simulink library "inp"  (R2021b)
settings: Solver=VariableStepAuto  StartTime=0.0  StopTime=10.0  RelTol=1e-3
undefined symbols (not defined in the file): C_TASK_5MS_S, FALSE, KINP_AcoreReadyToSlp_flg_ovrdflg, KINP_AcoreReadyToSlp_flg_ovrdval, KINP_AllowMovThd_OTA_enum_ovrdflg, KINP_AllowMovThd_OTA_enum_ovrdval, KINP_APSAngleTarget_Deg_ovrdflg, KINP_APSAngleTarget_Deg_ovrdval, KINP_APSDecReq_mps2_ovrdflg, KINP_APSDecReq_mps2_ovrdval, KINP_APSDecReqA_flg_ovrdflg, KINP_APSDecReqA_flg_ovrdval, KINP_APSDFLL_cm_ovrdflg, KINP_APSDFLL_cm_ovrdval, KINP_APSDFLR_cm_ovrdflg, KINP_APSDFLR_cm_ovrdval, KINP_APSDRLL_cm_ovrdflg, KINP_APSDRLL_cm_ovrdval, KINP_APSDRLR_cm_ovrdflg, KINP_APSDRLR_cm_ovrdval, KINP_APSExitCondition_enum_ovrdflg, KINP_APSExitCondition_enum_ovrdval, KINP_APSHWVer_enum_ovrdflg, KINP_APSHWVer_enum_ovrdval, KINP_APSProgressPCT_pct_ovrdflg, KINP_APSProgressPCT_pct_ovrdval, KINP_APSReq_enum_ovrdflg, KINP_APSReq_enum_ovrdval, KINP_APSRQDisplay_enum_ovrdflg, KINP_APSRQDisplay_enum_ovrdval, KINP_APSRqEPASCtrl_flg_ovrdflg, KINP_APSRqEPASCtrl_flg_ovrdval, KINP_APSShiftPosnReq_enum_ovrdval, KINP_APSShiftPosnReq_enum_ovrflg, KINP_APSSpeedCMD_kph_ovrdval, KINP_APSSpeedCMD_kph_ovrflg, KINP_APSStaSystem_enum_ovrdflg, KINP_APSStaSystem_enum_ovrdval, KINP_APSSWVer_enum_ovrdflg, KINP_APSSWVer_enum_ovrdval, KINP_APSVMCReqA_flg_ovrdval, KINP_APSVMCReqA_flg_ovrflg, KINP_APSVRqEPASCtrl_flg_ovrdflg, KINP_APSVRqEPASCtrl_flg_ovrdval, KINP_AuxBattVolmV_mV_ovrdflg, KINP_AuxBattVolmV_mV_ovrdval, KINP_CAASSta_enum_ovrdflg, KINP_CAASSta_enum_ovrdval, KINP_CAASVMCReqA_flg_ovrdval, KINP_CAASVMCReqA_flg_ovrflg, KINP_Chime_enum_ovrdflg, KINP_Chime_enum_ovrdval, KINP_ClearDTCcmd_flg_ovrdflg, KINP_ClearDTCcmd_flg_ovrdval, KINP_EvccAplusPwrUpReq_flg_ovrdflg, KINP_EvccAplusPwrUpReq_flg_ovrdval, KINP_LFID_raw_ovrdval, KINP_LFID_raw_ovrflg, KINP_LRID_raw_ovrdval, KINP_MemOffsetAccX_raw16_ovrdflg ... (+118)
libraries: FVT_lib x942, hcu_lib x1
(part 4 of 31)

== system inp/INP/CAN2/CreateBus ==
  inp_CanValid_bus : Inport
  inp_Hal_bus : Inport  Port=2
  UnitConverter_{1..19,22..28,31,35,43..46,49..50,54,56..59,61,64,70..71,75..77,81,88,91..92,95..102,107..108,113,115..116,119..121,123,125,127..128,130,133..136,147,149,151,154,156..157,159,161,164,166} (85 alike) : DataTypeConversion  OutDataTypeStr=boolean
  UnitConverter_{37..42,48,65,103..106,109,117..118,122,137..142,144..145,168..169,171..172} (28 alike) : DataTypeConversion  OutDataTypeStr=single
  UnitConverter_{20..21,29..30,32..34,36,47,51..53,55,60,62..63,67..69,72..74,78..80,82..87,89..90,93..94,110..112,114,124,126,129,131..132,143,146,148,150,152..153,155,158,160,162..163,165,167,170} (58 alike) : DataTypeConversion  OutDataTypeStr=uint8
  UnitConverter_66 : DataTypeConversion  OutDataTypeStr=uint32
  bus_creator : BusCreator  Inputs=172
  bus_selector : BusSelector  OutputSignals=VINP_CANMsgValidHMI1_flg,VINP_CANMsgValidIVI1_flg,VINP_CANMsgValidIVI2_flg,VINP_CANMsgValidIVI3_flg,VINP_CANMsgValidMETER1_flg
  bus_selector_1 : BusSelector  OutputSignals=VINP_HMIACAirIntMCmd_flg,VINP_HMIACAirIntPCmd_flg,VINP_HMIACAutoBtnCmd_flg,VINP_HMIACBtnCmd_flg,VINP_HMIACFrDefogBtnCmd_flg,VINP_HMIACRecycleBtnCmd_flg,VINP_HMIACWindDirMCmd_flg,VINP_HMIACWindDirPCmd_flg,VINP_HMIZ1SetTMCmd_flg,VINP_HMIZ1SetTPCmd_flg,VINP_HMIZ2SetTMCmd_flg,VINP_HMIZ2SetTPCmd_flg,VINP_AmbLighLowBatAlertSW_flg,VINP_AmbLighSafetyAlertSW_flg,VINP_AmbLightBrightnessSet_enum,VINP_AmbLightColorSet_enum,VINP_AmbLightDimInDarkSW_flg,VINP_AmbLightSW_flg,VINP_AmbLightWlcmLightSW_flg,VINP_FCPFrEvtBtnACMaxReq_flg,VINP_FCPFrEvtBtnACReq_flg,VINP_FCPFrEvtBtnAutoReq_flg,VINP_FCPFrEvtBtnSyncReq_flg,VINP_IVICreateAccReqSta_enum,VINP_IVIDelAccReqSta_enum,VINP_IVILinkAccReqSta_flg,VINP_IVILinkAccSta_enum,VINP_IVILinkKeySta_enum,VINP_IVILocatedSTA_enum,VINP_IVILockSoundSWSta_flg,VINP_IVITimeCheck_enum,VINP_IVITimeDay_DAY,VINP_IVITimeHour_hr,VINP_IVITimeMinute_min,VINP_IVITimeMonth_MONTH,VINP_IVITimeSecond_s,VINP_IVITimeYear_YEAR,VINP_LINKtoDrive_flg,VINP_OpenDrOpenWdoSW_flg,VINP_PWCONTINUEUSE_flg,VINP_SmartEcoModeSW_flg,VINP_UserSet_enum,VINP_ACChgCurSet_A,VINP_AVMErrSTA_flg,VINP_AVMOFFRecButt_flg,VINP_AVMParkingmode_enum,VINP_AVMparkingcancel_enum,VINP_AVMparkingexcute_enum,VINP_ApproachUnlockSW_flg,VINP_CAASSw_enum,VINP_CDLLockButt_flg,VINP_CDLUnlockButt_flg,VINP_DSEATantiset_flg,VINP_DSEATentryfunset_flg,VINP_DSEATventreq_enum,VINP_Distanceunit_flg,VINP_ESCSWCmd_enum,VINP_FSOffSw_enum,VINP_FollowMeSW_flg,VINP_GPSLAT_s,VINP_GPSLONG_enum,VINP_HeadLampSW_enum,VINP_HoodLatchSW_enum,VINP_IVIAirIntZ3Cmd_enum,VINP_IVIChargePortSWSta_flg,VINP_IVICreepSWReq_flg,VINP_IVIDSEATHeaterCmd_enum,VINP_IVIDSEATFroEdgeHeightCmd_enum,VINP_IVIDSEATHeightCmd_enum,VINP_IVIDSEATMemory1Sta_flg,VINP_IVIDSEATMemory2Sta_flg,VINP_IVIDSEATMemoryOPTCLSSta_flg,VINP_IVIDSEATReclineCmd_enum,VINP_IVIDSEATSlideCmd_enum,VINP_IVIISAOffsetSpd_enum,VINP_IVINightModeSta_flg,VINP_IVIPSEATHeaterCmd_enum,VINP_IVIPSEATReclineCmd_enum,VINP_IVIPSEATSlideCmd_enum,VINP_IVIPTGModeSW_enum,VINP_IVIPTGOpenHeight_enum,VINP_IVIPTGStaSW_enum,VINP_IVIPTGUSStaSW_flg,VINP_IVIPWModeReq_enum,VINP_IVIPwrLockSW_enum,VINP_IVIPwroffreq_flg,VINP_IVIRRDefReq_flg,VINP_IVIReqV2L_enum,VINP_IVIScreen_enum,VINP_IVIStartChgreq_flg,VINP_IVIStatus_flg,VINP_IVIStopChgreq_flg,VINP_IVITrailerCheckReqSta_flg,VINP_IVITrailerModeSWSta_flg,VINP_IVITriggerreq_flg,VINP_IVIUnlockChgreq_flg,VINP_IVIWIMAINSW_flg,VINP_LDrvControlCommand_pct,VINP_LPasControlCommand_pct,VINP_LRLDControlCommand_pct,VINP_LRRDControlCommand_pct,VINP_LightShowStartReq_flg,VINP_LightShowStopReq_flg,VINP_MFRDNBrightReq_pct,VINP_OFFACMODE_enum,VINP_PSEATventreq_enum,VINP_PerdV2L_enum,VINP_RFogLampSW_flg,VINP_RollModeSWCmd_enum,VINP_RoomLampMode_flg,VINP_SOCADJBUTT_flg,VINP_SOCLimitSet_pct,VINP_SOCV2LLimit_pct,VINP_SchedChgStart_flg,VINP_SchedChgStop_flg,VINP_SchedChgbutt_flg,VINP_SchedChglimit_pct,VINP_SchedChgwake_flg,VINP_SenstivityPosition_enum,VINP_SetUnlockSingle_flg,VINP_TCSSWCmd_enum,VINP_TPMSCaliButt_flg,VINP_TPMSResButt_flg,VINP_TurnSwTimeSet_enum,VINP_WalkawayLockSW_flg,VINP_WlcmLightMode_enum,VINP_sigAirIntenZon1Req_enum,VINP_sigDfrstReq_flg,VINP_sigFaceReq_flg,VINP_sigFootReq_flg,VINP_sigRecircReq_flg,VINP_sigSetTempZon1Req_C,VINP_sigSetTempZon2Req_C,VINP_IVICLBlowerYSta_pct,VINP_IVICLBlowerZSta_pct,VINP_IVICRBlowerYSta_pct,VINP_IVICRBlowerZSta_pct,VINP_IVIDrBlowerModeSta_enum,VINP_IVIDrBlowerYSta_pct,VINP_IVIDrBlowerZSta_pct,VINP_IVILSEATventCmd_enum,VINP_IVIMLFMostCmd_flg,VINP_IVIMLFootLiftCmd_enum,VINP_IVIMLNapModeCmd_flg,VINP_IVIMLReclinerCmd_enum,VINP_IVIMLRestoreCmd_flg,VINP_IVIMLSEATventCmd_enum,VINP_IVIMLSeatLiftCmd_enum,VINP_IVIMLSldRestoreCmd_flg,VINP_IVIMLSliderCmd_enum,VINP_IVIMLZeroGravityCmd_flg,VINP_IVIMRFMostCmd_flg,VINP_IVIMRFootLiftCmd_enum,VINP_IVIMRNapModeCmd_flg,VINP_IVIMRReclinerCmd_enum,VINP_IVIMRRestoreCmd_flg,VINP_IVIMRSEATventCmd_enum,VINP_IVIMRSeatLiftCmd_enum,VINP_IVIMRSldRestoreCmd_flg,VINP_IVIMRSliderCmd_enum,VINP_IVIMRZeroGravityCmd_flg,VINP_IVIPsBlowerModeSta_enum,VINP_IVIPsBlowerYSta_pct,VINP_IVIPsBlowerZSta_pct,VINP_IVIRSEATventCmd_enum,VINP_METERKPHCalcu_kph,VINP_ODOMETER_km
  BINP_outputs : Outport
  wires:
  inp_CanValid_bus/1 -> [inp_CanValid_bus]
  inp_Hal_bus/1 -> [inp_Hal_bus]
  bus_selector/1 -> UnitConverter_1/1  "<VINP_CANMsgValidHMI1_flg>"
  UnitConverter_1/1 -> bus_creator/1  "VINP_CANMsgValidHMI1_flg"
  bus_selector/2 -> UnitConverter_2/1  "<VINP_CANMsgValidIVI1_flg>"
  UnitConverter_2/1 -> bus_creator/2  "VINP_CANMsgValidIVI1_flg"
  bus_selector/3 -> UnitConverter_3/1  "<VINP_CANMsgValidIVI2_flg>"
  UnitConverter_3/1 -> bus_creator/3  "VINP_CANMsgValidIVI2_flg"
  bus_selector/4 -> UnitConverter_4/1  "<VINP_CANMsgValidIVI3_flg>"
  UnitConverter_4/1 -> bus_creator/4  "VINP_CANMsgValidIVI3_flg"
  bus_selector/5 -> UnitConverter_5/1  "<VINP_CANMsgValidMETER1_flg>"
  UnitConverter_5/1 -> bus_creator/5  "VINP_CANMsgValidMETER1_flg"
  bus_selector_1/1 -> UnitConverter_6/1  "<VINP_HMIACAirIntMCmd_flg>"
  UnitConverter_6/1 -> bus_creator/6  "VINP_HMIACAirIntMCmd_flg"
  bus_selector_1/2 -> UnitConverter_7/1  "<VINP_HMIACAirIntPCmd_flg>"
  UnitConverter_7/1 -> bus_creator/7  "VINP_HMIACAirIntPCmd_flg"
  bus_selector_1/3 -> UnitConverter_8/1  "<VINP_HMIACAutoBtnCmd_flg>"
  UnitConverter_8/1 -> bus_creator/8  "VINP_HMIACAutoBtnCmd_flg"
  bus_selector_1/4 -> UnitConverter_9/1  "<VINP_HMIACBtnCmd_flg>"
  UnitConverter_9/1 -> bus_creator/9  "VINP_HMIACBtnCmd_flg"
  bus_selector_1/5 -> UnitConverter_10/1  "<VINP_HMIACFrDefogBtnCmd_flg>"
  UnitConverter_10/1 -> bus_creator/10  "VINP_HMIACFrDefogBtnCmd_flg"
  bus_selector_1/6 -> UnitConverter_11/1  "<VINP_HMIACRecycleBtnCmd_flg>"
  UnitConverter_11/1 -> bus_creator/11  "VINP_HMIACRecycleBtnCmd_flg"
  bus_selector_1/7 -> UnitConverter_12/1  "<VINP_HMIACWindDirMCmd_flg>"
  UnitConverter_12/1 -> bus_creator/12  "VINP_HMIACWindDirMCmd_flg"
  bus_selector_1/8 -> UnitConverter_13/1  "<VINP_HMIACWindDirPCmd_flg>"
  UnitConverter_13/1 -> bus_creator/13  "VINP_HMIACWindDirPCmd_flg"
  bus_selector_1/9 -> UnitConverter_14/1  "<VINP_HMIZ1SetTMCmd_flg>"
  UnitConverter_14/1 -> bus_creator/14  "VINP_HMIZ1SetTMCmd_flg"
  bus_selector_1/10 -> UnitConverter_15/1  "<VINP_HMIZ1SetTPCmd_flg>"
  UnitConverter_15/1 -> bus_creator/15  "VINP_HMIZ1SetTPCmd_flg"
  bus_selector_1/11 -> UnitConverter_16/1  "<VINP_HMIZ2SetTMCmd_flg>"
  UnitConverter_16/1 -> bus_creator/16  "VINP_HMIZ2SetTMCmd_flg"
  bus_selector_1/12 -> UnitConverter_17/1  "<VINP_HMIZ2SetTPCmd_flg>"
  UnitConverter_17/1 -> bus_creator/17  "VINP_HMIZ2SetTPCmd_flg"
  bus_selector_1/13 -> UnitConverter_18/1  "<VINP_AmbLighLowBatAlertSW_flg>"
  UnitConverter_18/1 -> bus_creator/18  "VINP_AmbLighLowBatAlertSW_flg"
  bus_selector_1/14 -> UnitConverter_19/1  "<VINP_AmbLighSafetyAlertSW_flg>"
  UnitConverter_19/1 -> bus_creator/19  "VINP_AmbLighSafetyAlertSW_flg"
  bus_selector_1/15 -> UnitConverter_20/1  "<VINP_AmbLightBrightnessSet_enum>"
  UnitConverter_20/1 -> bus_creator/20  "VINP_AmbLightBrightnessSet_enum"
  bus_selector_1/16 -> UnitConverter_21/1  "<VINP_AmbLightColorSet_enum>"
  UnitConverter_21/1 -> bus_creator/21  "VINP_AmbLightColorSet_enum"
  bus_selector_1/17 -> UnitConverter_22/1  "<VINP_AmbLightDimInDarkSW_flg>"
  UnitConverter_22/1 -> bus_creator/22  "VINP_AmbLightDimInDarkSW_flg"
  bus_selector_1/18 -> UnitConverter_23/1  "<VINP_AmbLightSW_flg>"
  UnitConverter_23/1 -> bus_creator/23  "VINP_AmbLightSW_flg"
  bus_selector_1/19 -> UnitConverter_24/1  "<VINP_AmbLightWlcmLightSW_flg>"
  UnitConverter_24/1 -> bus_creator/24  "VINP_AmbLightWlcmLightSW_flg"
  bus_selector_1/20 -> UnitConverter_25/1  "<VINP_FCPFrEvtBtnACMaxReq_flg>"
  UnitConverter_25/1 -> bus_creator/25  "VINP_FCPFrEvtBtnACMaxReq_flg"
  bus_selector_1/21 -> UnitConverter_26/1  "<VINP_FCPFrEvtBtnACReq_flg>"
  UnitConverter_26/1 -> bus_creator/26  "VINP_FCPFrEvtBtnACReq_flg"
  bus_selector_1/22 -> UnitConverter_27/1  "<VINP_FCPFrEvtBtnAutoReq_flg>"
  UnitConverter_27/1 -> bus_creator/27  "VINP_FCPFrEvtBtnAutoReq_flg"
  bus_selector_1/23 -> UnitConverter_28/1  "<VINP_FCPFrEvtBtnSyncReq_flg>"
  UnitConverter_28/1 -> bus_creator/28  "VINP_FCPFrEvtBtnSyncReq_flg"
  bus_selector_1/24 -> UnitConverter_29/1  "<VINP_IVICreateAccReqSta_enum>"
  UnitConverter_29/1 -> bus_creator/29  "VINP_IVICreateAccReqSta_enum"
  bus_selector_1/25 -> UnitConverter_30/1  "<VINP_IVIDelAccReqSta_enum>"
  UnitConverter_30/1 -> bus_creator/30  "VINP_IVIDelAccReqSta_enum"
  bus_selector_1/26 -> UnitConverter_31/1  "<VINP_IVILinkAccReqSta_flg>"
  UnitConverter_31/1 -> bus_creator/31  "VINP_IVILinkAccReqSta_flg"
  bus_selector_1/27 -> UnitConverter_32/1  "<VINP_IVILinkAccSta_enum>"
  UnitConverter_32/1 -> bus_creator/32  "VINP_IVILinkAccSta_enum"
  bus_selector_1/28 -> UnitConverter_33/1  "<VINP_IVILinkKeySta_enum>"
  UnitConverter_33/1 -> bus_creator/33  "VINP_IVILinkKeySta_enum"
  bus_selector_1/29 -> UnitConverter_34/1  "<VINP_IVILocatedSTA_enum>"
  UnitConverter_34/1 -> bus_creator/34  "VINP_IVILocatedSTA_enum"
  bus_selector_1/30 -> UnitConverter_35/1  "<VINP_IVILockSoundSWSta_flg>"
  UnitConverter_35/1 -> bus_creator/35  "VINP_IVILockSoundSWSta_flg"
  bus_selector_1/31 -> UnitConverter_36/1  "<VINP_IVITimeCheck_enum>"
  UnitConverter_36/1 -> bus_creator/36  "VINP_IVITimeCheck_enum"
  bus_selector_1/32 -> UnitConverter_37/1  "<VINP_IVITimeDay_DAY>"
  UnitConverter_37/1 -> bus_creator/37  "VINP_IVITimeDay_DAY"
  bus_selector_1/33 -> UnitConverter_38/1  "<VINP_IVITimeHour_hr>"
  UnitConverter_38/1 -> bus_creator/38  "VINP_IVITimeHour_hr"
  bus_selector_1/34 -> UnitConverter_39/1  "<VINP_IVITimeMinute_min>"
  UnitConverter_39/1 -> bus_creator/39  "VINP_IVITimeMinute_min"
  bus_selector_1/35 -> UnitConverter_40/1  "<VINP_IVITimeMonth_MONTH>"
  UnitConverter_40/1 -> bus_creator/40  "VINP_IVITimeMonth_MONTH"
  bus_selector_1/36 -> UnitConverter_41/1  "<VINP_IVITimeSecond_s>"
  UnitConverter_41/1 -> bus_creator/41  "VINP_IVITimeSecond_s"
  bus_selector_1/37 -> UnitConverter_42/1  "<VINP_IVITimeYear_YEAR>"
  UnitConverter_42/1 -> bus_creator/42  "VINP_IVITimeYear_YEAR"
  bus_selector_1/38 -> UnitConverter_43/1  "<VINP_LINKtoDrive_flg>"
  UnitConverter_43/1 -> bus_creator/43  "VINP_LINKtoDrive_flg"
  bus_selector_1/39 -> UnitConverter_44/1  "<VINP_OpenDrOpenWdoSW_flg>"
  UnitConverter_44/1 -> bus_creator/44  "VINP_OpenDrOpenWdoSW_flg"
  bus_selector_1/40 -> UnitConverter_45/1  "<VINP_PWCONTINUEUSE_flg>"
  UnitConverter_45/1 -> bus_creator/45  "VINP_PWCONTINUEUSE_flg"
  bus_selector_1/41 -> UnitConverter_46/1  "<VINP_SmartEcoModeSW_flg>"
  UnitConverter_46/1 -> bus_creator/46  "VINP_SmartEcoModeSW_flg"
  bus_selector_1/42 -> UnitConverter_47/1  "<VINP_UserSet_enum>"
  UnitConverter_47/1 -> bus_creator/47  "VINP_UserSet_enum"
  bus_selector_1/43 -> UnitConverter_48/1  "<VINP_ACChgCurSet_A>"
  UnitConverter_48/1 -> bus_creator/48  "VINP_ACChgCurSet_A"
  bus_selector_1/44 -> UnitConverter_49/1  "<VINP_AVMErrSTA_flg>"
  UnitConverter_49/1 -> bus_creator/49  "VINP_AVMErrSTA_flg"
  bus_selector_1/45 -> UnitConverter_50/1  "<VINP_AVMOFFRecButt_flg>"
  UnitConverter_50/1 -> bus_creator/50  "VINP_AVMOFFRecButt_flg"
  bus_selector_1/46 -> UnitConverter_51/1  "<VINP_AVMParkingmode_enum>"
  UnitConverter_51/1 -> bus_creator/51  "VINP_AVMParkingmode_enum"
  bus_selector_1/47 -> UnitConverter_52/1  "<VINP_AVMparkingcancel_enum>"
  UnitConverter_52/1 -> bus_creator/52  "VINP_AVMparkingcancel_enum"
  bus_selector_1/48 -> UnitConverter_53/1  "<VINP_AVMparkingexcute_enum>"
  UnitConverter_53/1 -> bus_creator/53  "VINP_AVMparkingexcute_enum"
  bus_selector_1/49 -> UnitConverter_54/1  "<VINP_ApproachUnlockSW_flg>"
  UnitConverter_54/1 -> bus_creator/54  "VINP_ApproachUnlockSW_flg"
  bus_selector_1/50 -> UnitConverter_55/1  "<VINP_CAASSw_enum>"
  UnitConverter_55/1 -> bus_creator/55  "VINP_CAASSw_enum"
  bus_selector_1/51 -> UnitConverter_56/1  "<VINP_CDLLockButt_flg>"
  UnitConverter_56/1 -> bus_creator/56  "VINP_CDLLockButt_flg"
  bus_selector_1/52 -> UnitConverter_57/1  "<VINP_CDLUnlockButt_flg>"
  UnitConverter_57/1 -> bus_creator/57  "VINP_CDLUnlockButt_flg"
  bus_selector_1/53 -> UnitConverter_58/1  "<VINP_DSEATantiset_flg>"
  UnitConverter_58/1 -> bus_creator/58  "VINP_DSEATantiset_flg"
  bus_selector_1/54 -> UnitConverter_59/1  "<VINP_DSEATentryfunset_flg>"
  UnitConverter_59/1 -> bus_creator/59  "VINP_DSEATentryfunset_flg"
  bus_selector_1/55 -> UnitConverter_60/1  "<VINP_DSEATventreq_enum>"
  UnitConverter_60/1 -> bus_creator/60  "VINP_DSEATventreq_enum"
  bus_selector_1/56 -> UnitConverter_61/1  "<VINP_Distanceunit_flg>"
  UnitConverter_61/1 -> bus_creator/61  "VINP_Distanceunit_flg"
  bus_selector_1/57 -> UnitConverter_62/1  "<VINP_ESCSWCmd_enum>"
  UnitConverter_62/1 -> bus_creator/62  "VINP_ESCSWCmd_enum"
  bus_selector_1/58 -> UnitConverter_63/1  "<VINP_FSOffSw_enum>"
  UnitConverter_63/1 -> bus_creator/63  "VINP_FSOffSw_enum"
  bus_selector_1/59 -> UnitConverter_64/1  "<VINP_FollowMeSW_flg>"
  UnitConverter_64/1 -> bus_creator/64  "VINP_FollowMeSW_flg"
  bus_selector_1/60 -> UnitConverter_65/1  "<VINP_GPSLAT_s>"
  UnitConverter_65/1 -> bus_creator/65  "VINP_GPSLAT_s"
  bus_selector_1/61 -> UnitConverter_66/1  "<VINP_GPSLONG_enum>"
  UnitConverter_66/1 -> bus_creator/66  "VINP_GPSLONG_enum"
  bus_selector_1/62 -> UnitConverter_67/1  "<VINP_HeadLampSW_enum>"
  UnitConverter_67/1 -> bus_creator/67  "VINP_HeadLampSW_enum"
  bus_selector_1/63 -> UnitConverter_68/1  "<VINP_HoodLatchSW_enum>"
  UnitConverter_68/1 -> bus_creator/68  "VINP_HoodLatchSW_enum"
  bus_selector_1/64 -> UnitConverter_69/1  "<VINP_IVIAirIntZ3Cmd_enum>"
  UnitConverter_69/1 -> bus_creator/69  "VINP_IVIAirIntZ3Cmd_enum"
  bus_selector_1/65 -> UnitConverter_70/1  "<VINP_IVIChargePortSWSta_flg>"
  UnitConverter_70/1 -> bus_creator/70  "VINP_IVIChargePortSWSta_flg"
  bus_selector_1/66 -> UnitConverter_71/1  "<VINP_IVICreepSWReq_flg>"
  UnitConverter_71/1 -> bus_creator/71  "VINP_IVICreepSWReq_flg"
  bus_selector_1/67 -> UnitConverter_72/1  "<VINP_IVIDSEATHeaterCmd_enum>"
  UnitConverter_72/1 -> bus_creator/72  "VINP_IVIDSEATHeaterCmd_enum"
  bus_selector_1/68 -> UnitConverter_73/1  "<VINP_IVIDSEATFroEdgeHeightCmd_enum>"
  UnitConverter_73/1 -> bus_creator/73  "VINP_IVIDSEATFroEdgeHeightCmd_enum"
  bus_selector_1/69 -> UnitConverter_74/1  "<VINP_IVIDSEATHeightCmd_enum>"
  UnitConverter_74/1 -> bus_creator/74  "VINP_IVIDSEATHeightCmd_enum"
  bus_selector_1/70 -> UnitConverter_75/1  "<VINP_IVIDSEATMemory1Sta_flg>"
  UnitConverter_75/1 -> bus_creator/75  "VINP_IVIDSEATMemory1Sta_flg"
  bus_selector_1/71 -> UnitConverter_76/1  "<VINP_IVIDSEATMemory2Sta_flg>"
  UnitConverter_76/1 -> bus_creator/76  "VINP_IVIDSEATMemory2Sta_flg"
  bus_selector_1/72 -> UnitConverter_77/1  "<VINP_IVIDSEATMemoryOPTCLSSta_flg>"
  UnitConverter_77/1 -> bus_creator/77  "VINP_IVIDSEATMemoryOPTCLSSta_flg"
  bus_selector_1/73 -> UnitConverter_78/1  "<VINP_IVIDSEATReclineCmd_enum>"
  UnitConverter_78/1 -> bus_creator/78  "VINP_IVIDSEATReclineCmd_enum"
  bus_selector_1/74 -> UnitConverter_79/1  "<VINP_IVIDSEATSlideCmd_enum>"
  UnitConverter_79/1 -> bus_creator/79  "VINP_IVIDSEATSlideCmd_enum"
  bus_selector_1/75 -> UnitConverter_80/1  "<VINP_IVIISAOffsetSpd_enum>"
  UnitConverter_80/1 -> bus_creator/80  "VINP_IVIISAOffsetSpd_enum"
  bus_selector_1/76 -> UnitConverter_81/1  "<VINP_IVINightModeSta_flg>"
  UnitConverter_81/1 -> bus_creator/81  "VINP_IVINightModeSta_flg"
  bus_selector_1/77 -> UnitConverter_82/1  "<VINP_IVIPSEATHeaterCmd_enum>"
  UnitConverter_82/1 -> bus_creator/82  "VINP_IVIPSEATHeaterCmd_enum"
  bus_selector_1/78 -> UnitConverter_83/1  "<VINP_IVIPSEATReclineCmd_enum>"
  UnitConverter_83/1 -> bus_creator/83  "VINP_IVIPSEATReclineCmd_enum"
  bus_selector_1/79 -> UnitConverter_84/1  "<VINP_IVIPSEATSlideCmd_enum>"
  UnitConverter_84/1 -> bus_creator/84  "VINP_IVIPSEATSlideCmd_enum"
  bus_selector_1/80 -> UnitConverter_85/1  "<VINP_IVIPTGModeSW_enum>"
  UnitConverter_85/1 -> bus_creator/85  "VINP_IVIPTGModeSW_enum"
  bus_selector_1/81 -> UnitConverter_86/1  "<VINP_IVIPTGOpenHeight_enum>"
  UnitConverter_86/1 -> bus_creator/86  "VINP_IVIPTGOpenHeight_enum"
  bus_selector_1/82 -> UnitConverter_87/1  "<VINP_IVIPTGStaSW_enum>"
  UnitConverter_87/1 -> bus_creator/87  "VINP_IVIPTGStaSW_enum"
  bus_selector_1/83 -> UnitConverter_88/1  "<VINP_IVIPTGUSStaSW_flg>"
  UnitConverter_88/1 -> bus_creator/88  "VINP_IVIPTGUSStaSW_flg"
  bus_selector_1/84 -> UnitConverter_89/1  "<VINP_IVIPWModeReq_enum>"
  UnitConverter_89/1 -> bus_creator/89  "VINP_IVIPWModeReq_enum"
  bus_selector_1/85 -> UnitConverter_90/1  "<VINP_IVIPwrLockSW_enum>"
  UnitConverter_90/1 -> bus_creator/90  "VINP_IVIPwrLockSW_enum"
  bus_selector_1/86 -> UnitConverter_91/1  "<VINP_IVIPwroffreq_flg>"
  UnitConverter_91/1 -> bus_creator/91  "VINP_IVIPwroffreq_flg"
  bus_selector_1/87 -> UnitConverter_92/1  "<VINP_IVIRRDefReq_flg>"
  UnitConverter_92/1 -> bus_creator/92  "VINP_IVIRRDefReq_flg"
  bus_selector_1/88 -> UnitConverter_93/1  "<VINP_IVIReqV2L_enum>"
  UnitConverter_93/1 -> bus_creator/93  "VINP_IVIReqV2L_enum"
  bus_selector_1/89 -> UnitConverter_94/1  "<VINP_IVIScreen_enum>"
  UnitConverter_94/1 -> bus_creator/94  "VINP_IVIScreen_enum"
  bus_selector_1/90 -> UnitConverter_95/1  "<VINP_IVIStartChgreq_flg>"
  UnitConverter_95/1 -> bus_creator/95  "VINP_IVIStartChgreq_flg"
  bus_selector_1/91 -> UnitConverter_96/1  "<VINP_IVIStatus_flg>"
  UnitConverter_96/1 -> bus_creator/96  "VINP_IVIStatus_flg"
  bus_selector_1/92 -> UnitConverter_97/1  "<VINP_IVIStopChgreq_flg>"
  UnitConverter_97/1 -> bus_creator/97  "VINP_IVIStopChgreq_flg"
  bus_selector_1/93 -> UnitConverter_98/1  "<VINP_IVITrailerCheckReqSta_flg>"
  UnitConverter_98/1 -> bus_creator/98  "VINP_IVITrailerCheckReqSta_flg"
  bus_selector_1/94 -> UnitConverter_99/1  "<VINP_IVITrailerModeSWSta_flg>"
  UnitConverter_99/1 -> bus_creator/99  "VINP_IVITrailerModeSWSta_flg"
  bus_selector_1/95 -> UnitConverter_100/1  "<VINP_IVITriggerreq_flg>"
  UnitConverter_100/1 -> bus_creator/100  "VINP_IVITriggerreq_flg"
  bus_selector_1/96 -> UnitConverter_101/1  "<VINP_IVIUnlockChgreq_flg>"
  UnitConverter_101/1 -> bus_creator/101  "VINP_IVIUnlockChgreq_flg"
  bus_selector_1/97 -> UnitConverter_102/1  "<VINP_IVIWIMAINSW_flg>"
  UnitConverter_102/1 -> bus_creator/102  "VINP_IVIWIMAINSW_flg"
  bus_selector_1/98 -> UnitConverter_103/1  "<VINP_LDrvControlCommand_pct>"
  UnitConverter_103/1 -> bus_creator/103  "VINP_LDrvControlCommand_pct"
  bus_selector_1/99 -> UnitConverter_104/1  "<VINP_LPasControlCommand_pct>"
  UnitConverter_104/1 -> bus_creator/104  "VINP_LPasControlCommand_pct"
  bus_selector_1/100 -> UnitConverter_105/1  "<VINP_LRLDControlCommand_pct>"
  UnitConverter_105/1 -> bus_creator/105  "VINP_LRLDControlCommand_pct"
  bus_selector_1/101 -> UnitConverter_106/1  "<VINP_LRRDControlCommand_pct>"
  UnitConverter_106/1 -> bus_creator/106  "VINP_LRRDControlCommand_pct"
  bus_selector_1/102 -> UnitConverter_107/1  "<VINP_LightShowStartReq_flg>"
  UnitConverter_107/1 -> bus_creator/107  "VINP_LightShowStartReq_flg"
  bus_selector_1/103 -> UnitConverter_108/1  "<VINP_LightShowStopReq_flg>"
  UnitConverter_108/1 -> bus_creator/108  "VINP_LightShowStopReq_flg"
  bus_selector_1/104 -> UnitConverter_109/1  "<VINP_MFRDNBrightReq_pct>"
  UnitConverter_109/1 -> bus_creator/109  "VINP_MFRDNBrightReq_pct"
  bus_selector_1/105 -> UnitConverter_110/1  "<VINP_OFFACMODE_enum>"
  UnitConverter_110/1 -> bus_creator/110  "VINP_OFFACMODE_enum"
  bus_selector_1/106 -> UnitConverter_111/1  "<VINP_PSEATventreq_enum>"
  UnitConverter_111/1 -> bus_creator/111  "VINP_PSEATventreq_enum"
  bus_selector_1/107 -> UnitConverter_112/1  "<VINP_PerdV2L_enum>"
  UnitConverter_112/1 -> bus_creator/112  "VINP_PerdV2L_enum"
  bus_selector_1/108 -> UnitConverter_113/1  "<VINP_RFogLampSW_flg>"
  UnitConverter_113/1 -> bus_creator/113  "VINP_RFogLampSW_flg"
  bus_selector_1/109 -> UnitConverter_114/1  "<VINP_RollModeSWCmd_enum>"
  UnitConverter_114/1 -> bus_creator/114  "VINP_RollModeSWCmd_enum"
  bus_selector_1/110 -> UnitConverter_115/1  "<VINP_RoomLampMode_flg>"
  UnitConverter_115/1 -> bus_creator/115  "VINP_RoomLampMode_flg"
  bus_selector_1/111 -> UnitConverter_116/1  "<VINP_SOCADJBUTT_flg>"
  UnitConverter_116/1 -> bus_creator/116  "VINP_SOCADJBUTT_flg"
  bus_selector_1/112 -> UnitConverter_117/1  "<VINP_SOCLimitSet_pct>"
  UnitConverter_117/1 -> bus_creator/117  "VINP_SOCLimitSet_pct"
  bus_selector_1/113 -> UnitConverter_118/1  "<VINP_SOCV2LLimit_pct>"
  UnitConverter_118/1 -> bus_creator/118  "VINP_SOCV2LLimit_pct"
  bus_selector_1/114 -> UnitConverter_119/1  "<VINP_SchedChgStart_flg>"
  UnitConverter_119/1 -> bus_creator/119  "VINP_SchedChgStart_flg"
  bus_selector_1/115 -> UnitConverter_120/1  "<VINP_SchedChgStop_flg>"
  UnitConverter_120/1 -> bus_creator/120  "VINP_SchedChgStop_flg"
  bus_selector_1/116 -> UnitConverter_121/1  "<VINP_SchedChgbutt_flg>"
  UnitConverter_121/1 -> bus_creator/121  "VINP_SchedChgbutt_flg"
  bus_selector_1/117 -> UnitConverter_122/1  "<VINP_SchedChglimit_pct>"
  UnitConverter_122/1 -> bus_creator/122  "VINP_SchedChglimit_pct"
  bus_selector_1/118 -> UnitConverter_123/1  "<VINP_SchedChgwake_flg>"
  UnitConverter_123/1 -> bus_creator/123  "VINP_SchedChgwake_flg"
  bus_selector_1/119 -> UnitConverter_124/1  "<VINP_SenstivityPosition_enum>"
  UnitConverter_124/1 -> bus_creator/124  "VINP_SenstivityPosition_enum"
  bus_selector_1/120 -> UnitConverter_125/1  "<VINP_SetUnlockSingle_flg>"
  UnitConverter_125/1 -> bus_creator/125  "VINP_SetUnlockSingle_flg"
  bus_selector_1/121 -> UnitConverter_126/1  "<VINP_TCSSWCmd_enum>"
  UnitConverter_126/1 -> bus_creator/126  "VINP_TCSSWCmd_enum"
  bus_selector_1/122 -> UnitConverter_127/1  "<VINP_TPMSCaliButt_flg>"
  UnitConverter_127/1 -> bus_creator/127  "VINP_TPMSCaliButt_flg"
  bus_selector_1/123 -> UnitConverter_128/1  "<VINP_TPMSResButt_flg>"
  UnitConverter_128/1 -> bus_creator/128  "VINP_TPMSResButt_flg"
  bus_selector_1/124 -> UnitConverter_129/1  "<VINP_TurnSwTimeSet_enum>"
  UnitConverter_129/1 -> bus_creator/129  "VINP_TurnSwTimeSet_enum"
  bus_selector_1/125 -> UnitConverter_130/1  "<VINP_WalkawayLockSW_flg>"
  UnitConverter_130/1 -> bus_creator/130  "VINP_WalkawayLockSW_flg"
  bus_selector_1/126 -> UnitConverter_131/1  "<VINP_WlcmLightMode_enum>"
  UnitConverter_131/1 -> bus_creator/131  "VINP_WlcmLightMode_enum"
  bus_selector_1/127 -> UnitConverter_132/1  "<VINP_sigAirIntenZon1Req_enum>"
  UnitConverter_132/1 -> bus_creator/132  "VINP_sigAirIntenZon1Req_enum"
  bus_selector_1/128 -> UnitConverter_133/1  "<VINP_sigDfrstReq_flg>"
  UnitConverter_133/1 -> bus_creator/133  "VINP_sigDfrstReq_flg"
  bus_selector_1/129 -> UnitConverter_134/1  "<VINP_sigFaceReq_flg>"
  UnitConverter_134/1 -> bus_creator/134  "VINP_sigFaceReq_flg"
  bus_selector_1/130 -> UnitConverter_135/1  "<VINP_sigFootReq_flg>"
  UnitConverter_135/1 -> bus_creator/135  "VINP_sigFootReq_flg"
  bus_selector_1/131 -> UnitConverter_136/1  "<VINP_sigRecircReq_flg>"
  UnitConverter_136/1 -> bus_creator/136  "VINP_sigRecircReq_flg"
  bus_selector_1/132 -> UnitConverter_137/1  "<VINP_sigSetTempZon1Req_C>"
  UnitConverter_137/1 -> bus_creator/137  "VINP_sigSetTempZon1Req_C"
  bus_selector_1/133 -> UnitConverter_138/1  "<VINP_sigSetTempZon2Req_C>"
  UnitConverter_138/1 -> bus_creator/138  "VINP_sigSetTempZon2Req_C"
  bus_selector_1/134 -> UnitConverter_139/1  "<VINP_IVICLBlowerYSta_pct>"
  UnitConverter_139/1 -> bus_creator/139  "VINP_IVICLBlowerYSta_pct"
  bus_selector_1/135 -> UnitConverter_140/1  "<VINP_IVICLBlowerZSta_pct>"
  UnitConverter_140/1 -> bus_creator/140  "VINP_IVICLBlowerZSta_pct"
  bus_selector_1/136 -> UnitConverter_141/1  "<VINP_IVICRBlowerYSta_pct>"
  UnitConverter_141/1 -> bus_creator/141  "VINP_IVICRBlowerYSta_pct"
  bus_selector_1/137 -> UnitConverter_142/1  "<VINP_IVICRBlowerZSta_pct>"
  UnitConverter_142/1 -> bus_creator/142  "VINP_IVICRBlowerZSta_pct"
  bus_selector_1/138 -> UnitConverter_143/1  "<VINP_IVIDrBlowerModeSta_enum>"
  UnitConverter_143/1 -> bus_creator/143  "VINP_IVIDrBlowerModeSta_enum"
  bus_selector_1/139 -> UnitConverter_144/1  "<VINP_IVIDrBlowerYSta_pct>"
  UnitConverter_144/1 -> bus_creator/144  "VINP_IVIDrBlowerYSta_pct"
  bus_selector_1/140 -> UnitConverter_145/1  "<VINP_IVIDrBlowerZSta_pct>"
  UnitConverter_145/1 -> bus_creator/145  "VINP_IVIDrBlowerZSta_pct"
  bus_selector_1/141 -> UnitConverter_146/1  "<VINP_IVILSEATventCmd_enum>"
  UnitConverter_146/1 -> bus_creator/146  "VINP_IVILSEATventCmd_enum"
  bus_selector_1/142 -> UnitConverter_147/1  "<VINP_IVIMLFMostCmd_flg>"
  UnitConverter_147/1 -> bus_creator/147  "VINP_IVIMLFMostCmd_flg"
  bus_selector_1/143 -> UnitConverter_148/1  "<VINP_IVIMLFootLiftCmd_enum>"
  UnitConverter_148/1 -> bus_creator/148  "VINP_IVIMLFootLiftCmd_enum"
  bus_selector_1/144 -> UnitConverter_149/1  "<VINP_IVIMLNapModeCmd_flg>"
  UnitConverter_149/1 -> bus_creator/149  "VINP_IVIMLNapModeCmd_flg"
  bus_selector_1/145 -> UnitConverter_150/1  "<VINP_IVIMLReclinerCmd_enum>"
  UnitConverter_150/1 -> bus_creator/150  "VINP_IVIMLReclinerCmd_enum"
  bus_selector_1/146 -> UnitConverter_151/1  "<VINP_IVIMLRestoreCmd_flg>"
  UnitConverter_151/1 -> bus_creator/151  "VINP_IVIMLRestoreCmd_flg"
  bus_selector_1/147 -> UnitConverter_152/1  "<VINP_IVIMLSEATventCmd_enum>"
  UnitConverter_152/1 -> bus_creator/152  "VINP_IVIMLSEATventCmd_enum"
  bus_selector_1/148 -> UnitConverter_153/1  "<VINP_IVIMLSeatLiftCmd_enum>"
  UnitConverter_153/1 -> bus_creator/153  "VINP_IVIMLSeatLiftCmd_enum"
  bus_selector_1/149 -> UnitConverter_154/1  "<VINP_IVIMLSldRestoreCmd_flg>"
  UnitConverter_154/1 -> bus_creator/154  "VINP_IVIMLSldRestoreCmd_flg"
  bus_selector_1/150 -> UnitConverter_155/1  "<VINP_IVIMLSliderCmd_enum>"
  UnitConverter_155/1 -> bus_creator/155  "VINP_IVIMLSliderCmd_enum"
  bus_selector_1/151 -> UnitConverter_156/1  "<VINP_IVIMLZeroGravityCmd_flg>"
  UnitConverter_156/1 -> bus_creator/156  "VINP_IVIMLZeroGravityCmd_flg"
  bus_selector_1/152 -> UnitConverter_157/1  "<VINP_IVIMRFMostCmd_flg>"
  UnitConverter_157/1 -> bus_creator/157  "VINP_IVIMRFMostCmd_flg"
  bus_selector_1/153 -> UnitConverter_158/1  "<VINP_IVIMRFootLiftCmd_enum>"
  UnitConverter_158/1 -> bus_creator/158  "VINP_IVIMRFootLiftCmd_enum"
  bus_selector_1/154 -> UnitConverter_159/1  "<VINP_IVIMRNapModeCmd_flg>"
  UnitConverter_159/1 -> bus_creator/159  "VINP_IVIMRNapModeCmd_flg"
  bus_selector_1/155 -> UnitConverter_160/1  "<VINP_IVIMRReclinerCmd_enum>"
  UnitConverter_160/1 -> bus_creator/160  "VINP_IVIMRReclinerCmd_enum"
  bus_selector_1/156 -> UnitConverter_161/1  "<VINP_IVIMRRestoreCmd_flg>"
  UnitConverter_161/1 -> bus_creator/161  "VINP_IVIMRRestoreCmd_flg"
  bus_selector_1/157 -> UnitConverter_162/1  "<VINP_IVIMRSEATventCmd_enum>"
  UnitConverter_162/1 -> bus_creator/162  "VINP_IVIMRSEATventCmd_enum"
  bus_selector_1/158 -> UnitConverter_163/1  "<VINP_IVIMRSeatLiftCmd_enum>"
  UnitConverter_163/1 -> bus_creator/163  "VINP_IVIMRSeatLiftCmd_enum"
  bus_selector_1/159 -> UnitConverter_164/1  "<VINP_IVIMRSldRestoreCmd_flg>"
  UnitConverter_164/1 -> bus_creator/164  "VINP_IVIMRSldRestoreCmd_flg"
  bus_selector_1/160 -> UnitConverter_165/1  "<VINP_IVIMRSliderCmd_enum>"
  UnitConverter_165/1 -> bus_creator/165  "VINP_IVIMRSliderCmd_enum"
  bus_selector_1/161 -> UnitConverter_166/1  "<VINP_IVIMRZeroGravityCmd_flg>"
  UnitConverter_166/1 -> bus_creator/166  "VINP_IVIMRZeroGravityCmd_flg"
  bus_selector_1/162 -> UnitConverter_167/1  "<VINP_IVIPsBlowerModeSta_enum>"
  UnitConverter_167/1 -> bus_creator/167  "VINP_IVIPsBlowerModeSta_enum"
  bus_selector_1/163 -> UnitConverter_168/1  "<VINP_IVIPsBlowerYSta_pct>"
  UnitConverter_168/1 -> bus_creator/168  "VINP_IVIPsBlowerYSta_pct"
  bus_selector_1/164 -> UnitConverter_169/1  "<VINP_IVIPsBlowerZSta_pct>"
  UnitConverter_169/1 -> bus_creator/169  "VINP_IVIPsBlowerZSta_pct"
  bus_selector_1/165 -> UnitConverter_170/1  "<VINP_IVIRSEATventCmd_enum>"
  UnitConverter_170/1 -> bus_creator/170  "VINP_IVIRSEATventCmd_enum"
  bus_selector_1/166 -> UnitConverter_171/1  "<VINP_METERKPHCalcu_kph>"
  UnitConverter_171/1 -> bus_creator/171  "VINP_METERKPHCalcu_kph"
  bus_selector_1/167 -> UnitConverter_172/1  "<VINP_ODOMETER_km>"
  UnitConverter_172/1 -> bus_creator/172  "VINP_ODOMETER_km"
  [inp_CanValid_bus] -> bus_selector/1
  [inp_Hal_bus] -> bus_selector_1/1
  bus_creator/1 -> BINP_outputs/1
